simulink model "SM_Offshore_Windturbine"  (R2021a)
settings: Solver=ode4  StartTime=0.0  StopTime=par.sym.Ttot  FixedStep=par.sym.max_dt  MaxStep=par.sym.max_dt  RelTol=1e-3
model workspace: external: MATLAB File C:\Users\d053704\Desktop\MOST\Structure\CAD\CAD_DataFile.m (data not in the file)
undefined symbols (not defined in the file): par, smiData, X, Y, Z
libraries: sm_lib x50, simulink_extras x29, vrlib x18, nesl_utility x10, dspstat3 x9, sharedutil x5, eeGeneralControl x2
(part 1 of 4)
settings Model: Creator=lorenzocottura  LastModifiedBy=d053704
settings SolverCC: AlgebraicLoopSolver=LineSearch
settings DataIOCC: ReturnWorkspaceOutputs=off  TimeSaveName=TIME
settings OptimizationCC: LifeSpan=inf
settings DebuggingCC: SFMachineParentedDataDiag=warning  ArithmeticOperatorsInVariantConditions=warning
settings SFSimCC: CustomCodeUndefinedFunction=UseInterfaceOnly
settings SimscapeCC: SimscapeNormalizeSystem=off

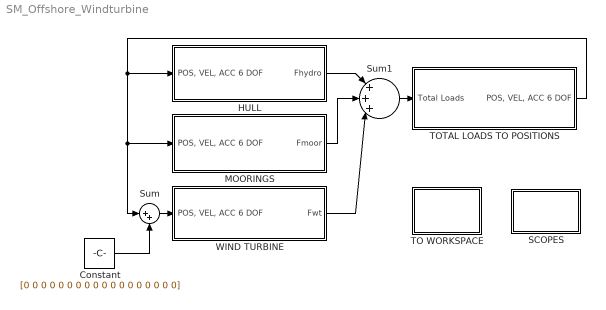
== system SM_Offshore_Windturbine ==
  Constant : Constant  Value=[0 0 0 0 0 0 0 0 0 0 0 0 0 0 0 0 0 0]
  HULL : Subsystem
  MOORINGS : Subsystem
  SCOPES : Subsystem
  Sum : Sum  Inputs=|++
  Sum1 : Sum  Inputs=|+++|
  TO WORKSPACE : Subsystem
  TOTAL LOADS TO POSITIONS : Subsystem
  WIND TURBINE : Subsystem
  wires:
  HULL/1(Fhydro) -> Sum1/1
  MOORINGS/1(Fmoor) -> Sum1/2
  WIND TURBINE/1(Fwt) -> Sum1/3
  Sum1/1 -> TOTAL LOADS TO POSITIONS/1(Total Loads)
  TOTAL LOADS TO POSITIONS/1("POS, VEL, ACC 6 DOF") -> HULL/1("POS, VEL, ACC 6 DOF"), Sum/1, MOORINGS/1("POS, VEL, ACC 6 DOF")
  Sum/1 -> WIND TURBINE/1("POS, VEL, ACC 6 DOF")
  Constant/1 -> Sum/2

== system SM_Offshore_Windturbine/HULL ==
  "POS, VEL, ACC 6 DOF" : Inport
  Add1 : Sum  Inputs=+-+-
  Hydrostatic stiffness : Subsystem
  IRR. WAVES : Subsystem
  Selector : Selector  InputPortWidth=18  IndexOptions=Index vector (dialog)  Indices=[1 2 3 4 5 6]  OutputSizes=1
  Selector1 : Selector  InputPortWidth=18  IndexOptions=Index vector (dialog)  Indices=[7 8 9 10 11 12]  OutputSizes=1
  State space model : Subsystem
  Viscous loads : Subsystem  TreatAsAtomicUnit=on
  Fhydro : Outport  VectorParamsAs1DForOutWhenUnconnected=off
  wires:
  Hydrostatic stiffness/1(Hydrostatic forces) -> Add1/2
  IRR. WAVES/1(Fw) -> Add1/1
  Selector1/1 -> State space model/1(hull_speed), Viscous loads/1(hull_speed)
  State space model/1(Radiation forces) -> Add1/4
  "POS, VEL, ACC 6 DOF"/1 -> Selector1/1, Selector/1
  Add1/1 -> Fhydro/1  "Hydrodinamic Loads"
  Viscous loads/1(Viscous forces) -> Add1/3
  Selector/1 -> Viscous loads/2(hull_position), Hydrostatic stiffness/1(hull_position)

== system SM_Offshore_Windturbine/MOORINGS ==
  "POS, VEL, ACC 6 DOF" : Inport
  6 Dof Extractor : Subsystem
  6 Dof Extractor1 : Subsystem
  6 Dof Extractor2 : Subsystem
  6 Dof Extractor3 : Subsystem
  6 Dof Extractor4 : Subsystem
  6 Dof Extractor5 : Subsystem
  Mux : Mux  Inputs=6
  n-D Lookup Table1 : Lookup_n-D  NumberOfTableDimensions=6  LookupTableObject=''  BreakpointsForDimension1=par.moor.LUT.x  BreakpointsForDimension2=par.moor.LUT.y  BreakpointsForDimension3=par.moor.LUT.z  BreakpointsForDimension4=par.moor.LUT.rx  BreakpointsForDimension5=par.moor.LUT.ry  BreakpointsForDimension6=par.moor.LUT.rz  BreakpointsForDimension1FirstPoint=10  BreakpointsForDimension2FirstPoint=10  BreakpointsForDimension1Spacing=12  BreakpointsForDimension2Spacing=12  Table=par.moor.LUT.Tx  TableDataTypeStr=Inherit: Inherit from 'Table data'  InternalRulePriority=Speed  RndMeth=Simplest  InputSameDT=on
      settings: InputPortMap=u0,u1,u2,u3,u4,u5
  n-D Lookup Table2 : Lookup_n-D  NumberOfTableDimensions=6  LookupTableObject=''  BreakpointsForDimension1=par.moor.LUT.x  BreakpointsForDimension2=par.moor.LUT.y  BreakpointsForDimension3=par.moor.LUT.z  BreakpointsForDimension4=par.moor.LUT.rx  BreakpointsForDimension5=par.moor.LUT.ry  BreakpointsForDimension6=par.moor.LUT.rz  BreakpointsForDimension1FirstPoint=10  BreakpointsForDimension2FirstPoint=10  BreakpointsForDimension1Spacing=12  BreakpointsForDimension2Spacing=12  Table=par.moor.LUT.Ty  TableDataTypeStr=Inherit: Inherit from 'Table data'  InternalRulePriority=Speed  RndMeth=Simplest  InputSameDT=on
      settings: InputPortMap=u0,u1,u2,u3,u4,u5
  n-D Lookup Table3 : Lookup_n-D  NumberOfTableDimensions=6  LookupTableObject=''  BreakpointsForDimension1=par.moor.LUT.x  BreakpointsForDimension2=par.moor.LUT.y  BreakpointsForDimension3=par.moor.LUT.z  BreakpointsForDimension4=par.moor.LUT.rx  BreakpointsForDimension5=par.moor.LUT.ry  BreakpointsForDimension6=par.moor.LUT.rz  BreakpointsForDimension1FirstPoint=10  BreakpointsForDimension2FirstPoint=10  BreakpointsForDimension1Spacing=12  BreakpointsForDimension2Spacing=12  Table=par.moor.LUT.Tz  TableDataTypeStr=Inherit: Inherit from 'Table data'  InternalRulePriority=Speed  RndMeth=Simplest  InputSameDT=on
      settings: InputPortMap=u0,u1,u2,u3,u4,u5
  n-D Lookup Table4 : Lookup_n-D  NumberOfTableDimensions=6  LookupTableObject=''  BreakpointsForDimension1=par.moor.LUT.x  BreakpointsForDimension2=par.moor.LUT.y  BreakpointsForDimension3=par.moor.LUT.z  BreakpointsForDimension4=par.moor.LUT.rx  BreakpointsForDimension5=par.moor.LUT.ry  BreakpointsForDimension6=par.moor.LUT.rz  BreakpointsForDimension1FirstPoint=10  BreakpointsForDimension2FirstPoint=10  BreakpointsForDimension1Spacing=12  BreakpointsForDimension2Spacing=12  Table=par.moor.LUT.TRx  TableDataTypeStr=Inherit: Inherit from 'Table data'  InternalRulePriority=Speed  RndMeth=Simplest  InputSameDT=on
      settings: InputPortMap=u0,u1,u2,u3,u4,u5
  n-D Lookup Table5 : Lookup_n-D  NumberOfTableDimensions=6  LookupTableObject=''  BreakpointsForDimension1=par.moor.LUT.x  BreakpointsForDimension2=par.moor.LUT.y  BreakpointsForDimension3=par.moor.LUT.z  BreakpointsForDimension4=par.moor.LUT.rx  BreakpointsForDimension5=par.moor.LUT.ry  BreakpointsForDimension6=par.moor.LUT.rz  BreakpointsForDimension1FirstPoint=10  BreakpointsForDimension2FirstPoint=10  BreakpointsForDimension1Spacing=12  BreakpointsForDimension2Spacing=12  Table=par.moor.LUT.TRy  TableDataTypeStr=Inherit: Inherit from 'Table data'  InternalRulePriority=Speed  RndMeth=Simplest  InputSameDT=on
      settings: InputPortMap=u0,u1,u2,u3,u4,u5
  n-D Lookup Table6 : Lookup_n-D  NumberOfTableDimensions=6  LookupTableObject=''  BreakpointsForDimension1=par.moor.LUT.x  BreakpointsForDimension2=par.moor.LUT.y  BreakpointsForDimension3=par.moor.LUT.z  BreakpointsForDimension4=par.moor.LUT.rx  BreakpointsForDimension5=par.moor.LUT.ry  BreakpointsForDimension6=par.moor.LUT.rz  BreakpointsForDimension1FirstPoint=10  BreakpointsForDimension2FirstPoint=10  BreakpointsForDimension1Spacing=12  BreakpointsForDimension2Spacing=12  Table=par.moor.LUT.TRz  TableDataTypeStr=Inherit: Inherit from 'Table data'  InternalRulePriority=Speed  RndMeth=Simplest  InputSameDT=on
      settings: InputPortMap=u0,u1,u2,u3,u4,u5
  Fmoor : Outport  VectorParamsAs1DForOutWhenUnconnected=off
  tag scope: MOORINGFORCES=global
  wires:
  6 Dof Extractor4/2(SWAY) -> n-D Lookup Table5/2
  n-D Lookup Table2/1 -> Mux/2  "Ty"
  6 Dof Extractor/2(SWAY) -> n-D Lookup Table1/2
  6 Dof Extractor3/6(YAW) -> n-D Lookup Table4/6
  n-D Lookup Table4/1 -> Mux/4  "TRx"
  6 Dof Extractor2/5(PITCH) -> n-D Lookup Table3/5
  6 Dof Extractor2/2(SWAY) -> n-D Lookup Table3/2
  6 Dof Extractor/1(SURGE) -> n-D Lookup Table1/1
  6 Dof Extractor5/6(YAW) -> n-D Lookup Table6/6
  n-D Lookup Table1/1 -> Mux/1  "Tx"
  6 Dof Extractor1/1(SURGE) -> n-D Lookup Table2/1
  n-D Lookup Table6/1 -> Mux/6  "TRz"
  6 Dof Extractor4/5(PITCH) -> n-D Lookup Table5/5
  6 Dof Extractor1/5(PITCH) -> n-D Lookup Table2/5
  6 Dof Extractor1/6(YAW) -> n-D Lookup Table2/6
  6 Dof Extractor2/6(YAW) -> n-D Lookup Table3/6
  6 Dof Extractor5/3(HEAVE) -> n-D Lookup Table6/3
  6 Dof Extractor/5(PITCH) -> n-D Lookup Table1/5
  n-D Lookup Table3/1 -> Mux/3  "Tz"
  6 Dof Extractor3/2(SWAY) -> n-D Lookup Table4/2
  6 Dof Extractor3/1(SURGE) -> n-D Lookup Table4/1
  6 Dof Extractor4/4(ROLL) -> n-D Lookup Table5/4
  6 Dof Extractor3/5(PITCH) -> n-D Lookup Table4/5
  6 Dof Extractor2/1(SURGE) -> n-D Lookup Table3/1
  6 Dof Extractor/4(ROLL) -> n-D Lookup Table1/4
  6 Dof Extractor3/4(ROLL) -> n-D Lookup Table4/4
  6 Dof Extractor1/2(SWAY) -> n-D Lookup Table2/2
  6 Dof Extractor/6(YAW) -> n-D Lookup Table1/6
  6 Dof Extractor1/4(ROLL) -> n-D Lookup Table2/4
  6 Dof Extractor5/4(ROLL) -> n-D Lookup Table6/4
  6 Dof Extractor1/3(HEAVE) -> n-D Lookup Table2/3
  6 Dof Extractor4/3(HEAVE) -> n-D Lookup Table5/3
  6 Dof Extractor2/4(ROLL) -> n-D Lookup Table3/4
  6 Dof Extractor4/1(SURGE) -> n-D Lookup Table5/1
  6 Dof Extractor3/3(HEAVE) -> n-D Lookup Table4/3
  6 Dof Extractor/3(HEAVE) -> n-D Lookup Table1/3
  6 Dof Extractor5/5(PITCH) -> n-D Lookup Table6/5
  6 Dof Extractor5/2(SWAY) -> n-D Lookup Table6/2
  n-D Lookup Table5/1 -> Mux/5  "TRy"
  6 Dof Extractor5/1(SURGE) -> n-D Lookup Table6/1
  6 Dof Extractor4/6(YAW) -> n-D Lookup Table5/6
  6 Dof Extractor2/3(HEAVE) -> n-D Lookup Table3/3
  Mux/1 -> Fmoor/1, [MOORINGFORCES]  "T_C"
  "POS, VEL, ACC 6 DOF"/1 -> 6 Dof Extractor4/1(6DOF), 6 Dof Extractor5/1(6DOF), 6 Dof Extractor3/1(6DOF), 6 Dof Extractor2/1(6DOF), 6 Dof Extractor1/1(6DOF), 6 Dof Extractor/1(6DOF)

== system SM_Offshore_Windturbine/SCOPES ==
  Divide1 : Product  Inputs=**
  GUIScopes : Scope  NumInputPorts=9
  Radians to Degrees4 : simulink_extras/Transformations/Radians to Degrees
  Radians to Degrees5 : simulink_extras/Transformations/Radians to Degrees
  Radians to Degrees6 : simulink_extras/Transformations/Radians to Degrees
  Selector{,1..5} (6 alike) : Selector  InputPortWidth=3  IndexOptions=Index vector (dialog)  Indices=[1]  OutputSizes=1
  W2MW1 : Gain  Gain=1e-6
  efficiency1 : Gain  Gain=0.944
  tag scope: GENPWR=global
  wires:
  [SURGE] -> Selector/1
  Selector/1 -> GUIScopes/1  "Surge [m]"
  [HEAVE] -> Selector1/1  "z"
  Selector1/1 -> GUIScopes/3  "Heave [m]"
  [SWAY] -> Selector2/1  "y"
  Selector2/1 -> GUIScopes/2  "Sway [m]"
  Radians to Degrees4/1 -> GUIScopes/4  "Roll [deg]"
  Radians to Degrees5/1 -> GUIScopes/5  "Pitch [deg]"
  Radians to Degrees6/1 -> GUIScopes/6  "Yaw [deg]"
  W2MW1/1 -> [GENPWR], GUIScopes/9  "Generator Power [MW]"
  [YAW] -> Selector4/1  "ry"
  Selector4/1 -> Radians to Degrees6/1
  Selector5/1 -> Radians to Degrees5/1
  Selector3/1 -> Radians to Degrees4/1
  [ROLL] -> Selector3/1  "ry"
  [PITCH] -> Selector5/1  "ry"
  [BlPITCH] -> GUIScopes/8  "Blade Pitch [deg]"
  [GENSPD] -> GUIScopes/7  "Generator Speed [rpm]"
  [Speed] -> Divide1/2
  [GENTRQ] -> Divide1/1  "GENTRQ"
  efficiency1/1 -> W2MW1/1
  Divide1/1 -> efficiency1/1

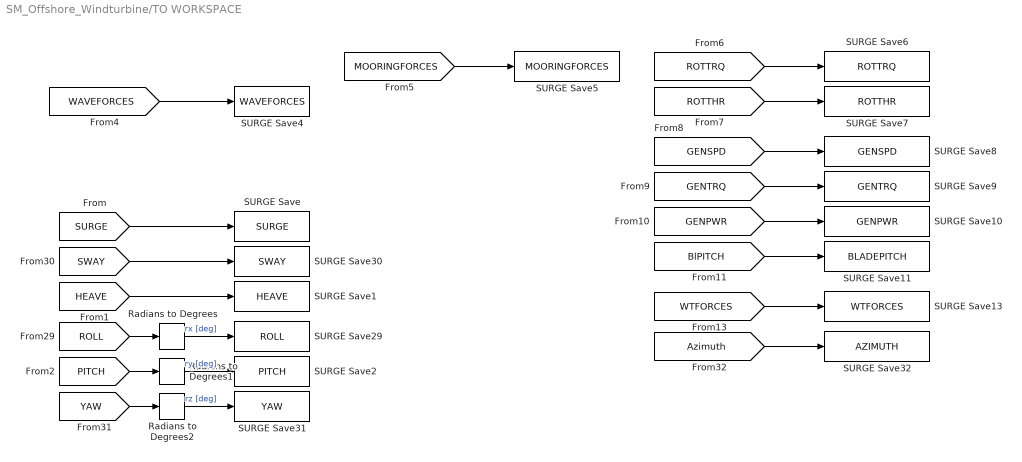
== system SM_Offshore_Windturbine/TO WORKSPACE ==
  Radians to Degrees : simulink_extras/Transformations/Radians to Degrees
  Radians to Degrees1 : simulink_extras/Transformations/Radians to Degrees
  Radians to Degrees2 : simulink_extras/Transformations/Radians to Degrees
  SURGE Save : ToWorkspace  VariableName=SURGE  SampleTime=-1
  SURGE Save1 : ToWorkspace  VariableName=HEAVE  SampleTime=-1
  SURGE Save10 : ToWorkspace  VariableName=GENPWR  SampleTime=-1
  SURGE Save11 : ToWorkspace  VariableName=BLADEPITCH  SampleTime=-1
  SURGE Save13 : ToWorkspace  VariableName=WTFORCES  SampleTime=-1
  SURGE Save2 : ToWorkspace  VariableName=PITCH  SampleTime=-1
  SURGE Save29 : ToWorkspace  VariableName=ROLL  SampleTime=-1
  SURGE Save30 : ToWorkspace  VariableName=SWAY  SampleTime=-1
  SURGE Save31 : ToWorkspace  VariableName=YAW  SampleTime=-1
  SURGE Save32 : ToWorkspace  VariableName=AZIMUTH  SampleTime=-1
  SURGE Save4 : ToWorkspace  VariableName=WAVEFORCES  SampleTime=-1
  SURGE Save5 : ToWorkspace  VariableName=MOORINGFORCES  SampleTime=-1
  SURGE Save6 : ToWorkspace  VariableName=ROTTRQ  SampleTime=-1
  SURGE Save7 : ToWorkspace  VariableName=ROTTHR  SampleTime=-1
  SURGE Save8 : ToWorkspace  VariableName=GENSPD  SampleTime=-1
  SURGE Save9 : ToWorkspace  VariableName=GENTRQ  SampleTime=-1
  wires:
  [SURGE] -> SURGE Save/1
  [HEAVE] -> SURGE Save1/1
  [PITCH] -> Radians to Degrees1/1
  [WAVEFORCES] -> SURGE Save4/1
  [MOORINGFORCES] -> SURGE Save5/1
  [ROTTRQ] -> SURGE Save6/1
  [ROTTHR] -> SURGE Save7/1
  [GENSPD] -> SURGE Save8/1
  [GENTRQ] -> SURGE Save9/1
  [GENPWR] -> SURGE Save10/1
  [BlPITCH] -> SURGE Save11/1
  [WTFORCES] -> SURGE Save13/1
  [ROLL] -> Radians to Degrees/1
  [YAW] -> Radians to Degrees2/1
  [SWAY] -> SURGE Save30/1
  [Azimuth] -> SURGE Save32/1
  Radians to Degrees/1 -> SURGE Save29/1  "rx [deg]"
  Radians to Degrees1/1 -> SURGE Save2/1  "ry [deg]"
  Radians to Degrees2/1 -> SURGE Save31/1  "rz [deg]"

== system SM_Offshore_Windturbine/TOTAL LOADS TO POSITIONS ==
  Total Loads : Inport
  "6 Dof Extractor TO SCOPES " : Subsystem
  Add : Sum  Inputs=-+-
  Added mass matrix : Constant  Value=par.hull.TDM.Ainf
  Gravity & Restoring moment : Subsystem
  Integrator : Integrator
  Integrator2 : Integrator
  Matrix Divide : Product  Inputs=/*  Multiplication=Matrix(*)
  Memory1 : Memory
  Memory2 : Memory
  Memory3 : Memory
  Mux : Mux  Inputs=3
  "Non linear loads " : Subsystem
  Sum : Sum
  Variable mass matrix1 : ModelReference  ModelNameDialog=Variable_mass_matrix.slxp  ModelReferenceVersion=5.19  CopyOfModelProtected=on
  "POS, VEL, ACC 6 DOF" : Outport  VectorParamsAs1DForOutWhenUnconnected=off
  wires:
  Integrator2/1 -> Memory2/1  "Position"
  Add/1 -> Matrix Divide/2
  Matrix Divide/1 -> Integrator/1, Memory3/1  "Acceleration"
  Variable mass matrix1/1 -> "Non linear loads "/1(MassMatrix), Sum/2, Gravity & Restoring moment/1(MassMatrix)
  "Non linear loads "/1(Non_linear) -> Add/3
  Mux/1 -> "POS, VEL, ACC 6 DOF"/1, "6 Dof Extractor TO SCOPES "/1(6DOF)
  Integrator/1 -> Integrator2/1, Memory1/1
  Memory2/1 -> Variable mass matrix1/1, Mux/1
  Memory1/1 -> "Non linear loads "/2(hull_speed), Mux/2
  Memory3/1 -> Mux/3
  Gravity & Restoring moment/1(Gravity & Restoring moment) -> Add/1
  Added mass matrix/1 -> Sum/1
  Sum/1 -> Matrix Divide/1
  Total Loads/1 -> Add/2

== system SM_Offshore_Windturbine/WIND TURBINE ==
  "POS, VEL, ACC 6 DOF" : Inport
  BODIES MOTIONS : Subsystem
  CONTROL SYSTEM : Subsystem
  N : Gain  Gain=par.WT.prop.Ngear
  "N " : Gain  Gain=par.WT.prop.Ngear
  ROTOR LOADS : Subsystem
  Fwt : Outport  VectorParamsAs1DForOutWhenUnconnected=off
  wires:
  ROTOR LOADS/1(WT Forces) -> Fwt/1
  CONTROL SYSTEM/1(Blade pitch) -> ROTOR LOADS/1(Blade pitch in), BODIES MOTIONS/1(Blade Pitch)
  CONTROL SYSTEM/3(Tg) -> "N "/1
  N/1 -> CONTROL SYSTEM/2(Generator speed)
  ROTOR LOADS/2(RotorTorque) -> BODIES MOTIONS/2(Rotor Torque)
  "N "/1 -> ROTOR LOADS/4(Control torque), BODIES MOTIONS/4(Control Torque)
  BODIES MOTIONS/1(Rotor Speed) -> ROTOR LOADS/2(Rotor speed), N/1
  "POS, VEL, ACC 6 DOF"/1 -> CONTROL SYSTEM/1(6 DOF)
  CONTROL SYSTEM/2(6 DOF nac) -> BODIES MOTIONS/3(6 DOF), ROTOR LOADS/3(6 DOF)
  ROTOR LOADS/3(Wind Direct) -> CONTROL SYSTEM/3(Wind direction)

== system SM_Offshore_Windturbine/HULL/Hydrostatic stiffness ==
  hull_position : Inport
  Constant : Constant  Value=[0 0 par.hull.GEOM.V0*par.hull.ENV.rho_w*9.80665 0 0 0]
  Hydrostatic stiffness : Constant  Value=par.hull.FDA.hydrostatic.K
  Product2 : Product  Multiplication=Matrix(*)  RndMeth=Zero
  Sum1 : Sum  Inputs=|+-
  Hydrostatic forces : Outport  VectorParamsAs1DForOutWhenUnconnected=off
  wires:
  Sum1/1 -> Hydrostatic forces/1
  Constant/1 -> Sum1/2
  Product2/1 -> Sum1/1
  Hydrostatic stiffness/1 -> Product2/1
  hull_position/1 -> Product2/2

== system SM_Offshore_Windturbine/HULL/IRR. WAVES ==
  Excitation forces : FromWorkspace  VariableName=[par.wave.TIME,par.wave.forces.TAU]
  Fw : Outport  VectorParamsAs1DForOutWhenUnconnected=off
  tag scope: WAVEFORCES=global
  wires:
  Excitation forces/1 -> [WAVEFORCES], Fw/1

== system SM_Offshore_Windturbine/HULL/State space model ==
  hull_speed : Inport
  Demux : Demux  Outputs=6
  Mux : Mux  Inputs=6
  State-Space1 : StateSpace  A=par.hull.TDM.(DOFs).Ass  B=par.hull.TDM.(DOFs).Bss  C=par.hull.TDM.(DOFs).Css  D=par.hull.TDM.(DOFs).Dss  InitialCondition=0  mask{DOFs='y'}
      mask prompts: DOFs "Degree of freedom selection (e.g. 'x_ry', 'x'; include apostrophes)"
      mask help:
      | State-space model:
      |    dx/dt = Ax + Bu
      |            y = Cx + Du
      mask Display:
      | color('black')
      | 
      | if isempty(findstr(DOFs,'_'))
      |     in = DOFs;
      | else
      |     in = DOFs(1:findstr(DOFs,'_')-1);
      | end
      | 
      | port_label('input',1,in)
      | port_label('output',1,['F_{r,', strrep(DOFs,'_','-'), '}'],'texmode','on')
      | 
      | 
      | disp(['x'' = Ax + Bu' 10 'y = Cx + Du'],'texmode','on')
      | % text(0.5, 0, DOFs, 'horizontalAlignment', 'center', 'verticalAlignment', 'bottom')
  State-Space10 : StateSpace  A=par.hull.TDM.(DOFs).Ass  B=par.hull.TDM.(DOFs).Bss  C=par.hull.TDM.(DOFs).Css  D=par.hull.TDM.(DOFs).Dss  InitialCondition=0  mask{DOFs='rz'}
      mask prompts: DOFs "Degree of freedom selection (e.g. 'x_ry', 'x'; include apostrophes)"
      mask help:
      | State-space model:
      |    dx/dt = Ax + Bu
      |            y = Cx + Du
      mask Display:
      | color('black')
      | 
      | if isempty(findstr(DOFs,'_'))
      |     in = DOFs;
      | else
      |     in = DOFs(1:findstr(DOFs,'_')-1);
      | end
      | 
      | port_label('input',1,in)
      | port_label('output',1,['F_{r,', strrep(DOFs,'_','-'), '}'],'texmode','on')
      | 
      | 
      | disp(['x'' = Ax + Bu' 10 'y = Cx + Du'],'texmode','on')
      | % text(0.5, 0, DOFs, 'horizontalAlignment', 'center', 'verticalAlignment', 'bottom')
  State-Space2 : StateSpace  A=par.hull.TDM.(DOFs).Ass  B=par.hull.TDM.(DOFs).Bss  C=par.hull.TDM.(DOFs).Css  D=par.hull.TDM.(DOFs).Dss  InitialCondition=0  mask{DOFs='x'}
      mask prompts: DOFs "Degree of freedom selection (e.g. 'x_ry', 'x'; include apostrophes)"
      mask help:
      | State-space model:
      |    dx/dt = Ax + Bu
      |            y = Cx + Du
      mask Display:
      | color('black')
      | 
      | if isempty(findstr(DOFs,'_'))
      |     in = DOFs;
      | else
      |     in = DOFs(1:findstr(DOFs,'_')-1);
      | end
      | 
      | port_label('input',1,in)
      | port_label('output',1,['F_{r,', strrep(DOFs,'_','-'), '}'],'texmode','on')
      | 
      | 
      | disp(['x'' = Ax + Bu' 10 'y = Cx + Du'],'texmode','on')
  State-Space3 : StateSpace  A=par.hull.TDM.(DOFs).Ass  B=par.hull.TDM.(DOFs).Bss  C=par.hull.TDM.(DOFs).Css  D=par.hull.TDM.(DOFs).Dss  InitialCondition=0  mask{DOFs='ry_x'}
      mask prompts: DOFs "Degree of freedom selection (e.g. 'x_ry', 'x'; include apostrophes)"
      mask help:
      | State-space model:
      |    dx/dt = Ax + Bu
      |            y = Cx + Du
      mask Display:
      | color('black')
      | 
      | if isempty(findstr(DOFs,'_'))
      |     in = DOFs;
      | else
      |     in = DOFs(1:findstr(DOFs,'_')-1);
      | end
      | 
      | port_label('input',1,in)
      | port_label('output',1,['F_{r,', strrep(DOFs,'_','-'), '}'],'texmode','on')
      | 
      | 
      | disp(['x'' = Ax + Bu' 10 'y = Cx + Du'],'texmode','on')
      | % text(0.5, 0, DOFs, 'horizontalAlignment', 'center', 'verticalAlignment', 'bottom')
  State-Space4 : StateSpace  A=par.hull.TDM.(DOFs).Ass  B=par.hull.TDM.(DOFs).Bss  C=par.hull.TDM.(DOFs).Css  D=par.hull.TDM.(DOFs).Dss  InitialCondition=0  mask{DOFs='rx'}
      mask prompts: DOFs "Degree of freedom selection (e.g. 'x_ry', 'x'; include apostrophes)"
      mask help:
      | State-space model:
      |    dx/dt = Ax + Bu
      |            y = Cx + Du
      mask Display:
      | color('black')
      | 
      | if isempty(findstr(DOFs,'_'))
      |     in = DOFs;
      | else
      |     in = DOFs(1:findstr(DOFs,'_')-1);
      | end
      | 
      | port_label('input',1,in)
      | port_label('output',1,['F_{r,', strrep(DOFs,'_','-'), '}'],'texmode','on')
      | 
      | 
      | disp(['x'' = Ax + Bu' 10 'y = Cx + Du'],'texmode','on')
      | % text(0.5, 0, DOFs, 'horizontalAlignment', 'center', 'verticalAlignment', 'bottom')
  State-Space5 : StateSpace  A=par.hull.TDM.(DOFs).Ass  B=par.hull.TDM.(DOFs).Bss  C=par.hull.TDM.(DOFs).Css  D=par.hull.TDM.(DOFs).Dss  InitialCondition=0  mask{DOFs='z'}
      mask prompts: DOFs "Degree of freedom selection (e.g. 'x_ry', 'x'; include apostrophes)"
      mask help:
      | State-space model:
      |    dx/dt = Ax + Bu
      |            y = Cx + Du
      mask Display:
      | color('black')
      | 
      | if isempty(findstr(DOFs,'_'))
      |     in = DOFs;
      | else
      |     in = DOFs(1:findstr(DOFs,'_')-1);
      | end
      | 
      | port_label('input',1,in)
      | port_label('output',1,['F_{r,', strrep(DOFs,'_','-'), '}'],'texmode','on')
      | 
      | 
      | disp(['x'' = Ax + Bu' 10 'y = Cx + Du'],'texmode','on')
      | % text(0.5, 0, DOFs, 'horizontalAlignment', 'center', 'verticalAlignment', 'bottom')
  State-Space6 : StateSpace  A=par.hull.TDM.(DOFs).Ass  B=par.hull.TDM.(DOFs).Bss  C=par.hull.TDM.(DOFs).Css  D=par.hull.TDM.(DOFs).Dss  InitialCondition=0  mask{DOFs='x_ry'}
      mask prompts: DOFs "Degree of freedom selection (e.g. 'x_ry', 'x'; include apostrophes)"
      mask help:
      | State-space model:
      |    dx/dt = Ax + Bu
      |            y = Cx + Du
      mask Display:
      | color('black')
      | 
      | if isempty(findstr(DOFs,'_'))
      |     in = DOFs;
      | else
      |     in = DOFs(1:findstr(DOFs,'_')-1);
      | end
      | 
      | port_label('input',1,in)
      | port_label('output',1,['F_{r,', strrep(DOFs,'_','-'), '}'],'texmode','on')
      | 
      | 
      | disp(['x'' = Ax + Bu' 10 'y = Cx + Du'],'texmode','on')
      | % text(0.5, 0, DOFs, 'horizontalAlignment', 'center', 'verticalAlignment', 'bottom')
  State-Space7 : StateSpace  A=par.hull.TDM.(DOFs).Ass  B=par.hull.TDM.(DOFs).Bss  C=par.hull.TDM.(DOFs).Css  D=par.hull.TDM.(DOFs).Dss  InitialCondition=0  mask{DOFs='rx_y'}
      mask prompts: DOFs "Degree of freedom selection (e.g. 'x_ry', 'x'; include apostrophes)"
      mask help:
      | State-space model:
      |    dx/dt = Ax + Bu
      |            y = Cx + Du
      mask Display:
      | color('black')
      | 
      | if isempty(findstr(DOFs,'_'))
      |     in = DOFs;
      | else
      |     in = DOFs(1:findstr(DOFs,'_')-1);
      | end
      | 
      | port_label('input',1,in)
      | port_label('output',1,['F_{r,', strrep(DOFs,'_','-'), '}'],'texmode','on')
      | 
      | 
      | disp(['x'' = Ax + Bu' 10 'y = Cx + Du'],'texmode','on')
      | % text(0.5, 0, DOFs, 'horizontalAlignment', 'center', 'verticalAlignment', 'bottom')
  State-Space8 : StateSpace  A=par.hull.TDM.(DOFs).Ass  B=par.hull.TDM.(DOFs).Bss  C=par.hull.TDM.(DOFs).Css  D=par.hull.TDM.(DOFs).Dss  InitialCondition=0  mask{DOFs='ry'}
      mask prompts: DOFs "Degree of freedom selection (e.g. 'x_ry', 'x'; include apostrophes)"
      mask help:
      | State-space model:
      |    dx/dt = Ax + Bu
      |            y = Cx + Du
      mask Display:
      | color('black')
      | 
      | if isempty(findstr(DOFs,'_'))
      |     in = DOFs;
      | else
      |     in = DOFs(1:findstr(DOFs,'_')-1);
      | end
      | 
      | port_label('input',1,in)
      | port_label('output',1,['F_{r,', strrep(DOFs,'_','-'), '}'],'texmode','on')
      | 
      | 
      | disp(['x'' = Ax + Bu' 10 'y = Cx + Du'],'texmode','on')
      | % text(0.5, 0, DOFs, 'horizontalAlignment', 'center', 'verticalAlignment', 'bottom')
  State-Space9 : StateSpace  A=par.hull.TDM.(DOFs).Ass  B=par.hull.TDM.(DOFs).Bss  C=par.hull.TDM.(DOFs).Css  D=par.hull.TDM.(DOFs).Dss  InitialCondition=0  mask{DOFs='y_rx'}
      mask prompts: DOFs "Degree of freedom selection (e.g. 'x_ry', 'x'; include apostrophes)"
      mask help:
      | State-space model:
      |    dx/dt = Ax + Bu
      |            y = Cx + Du
      mask Display:
      | color('black')
      | 
      | if isempty(findstr(DOFs,'_'))
      |     in = DOFs;
      | else
      |     in = DOFs(1:findstr(DOFs,'_')-1);
      | end
      | 
      | port_label('input',1,in)
      | port_label('output',1,['F_{r,', strrep(DOFs,'_','-'), '}'],'texmode','on')
      | 
      | 
      | disp(['x'' = Ax + Bu' 10 'y = Cx + Du'],'texmode','on')
      | % text(0.5, 0, DOFs, 'horizontalAlignment', 'center', 'verticalAlignment', 'bottom')
  Sum{,1..3} (4 alike) : Sum  Inputs=|++
  Radiation forces : Outport  VectorParamsAs1DForOutWhenUnconnected=off
  wires:
  Demux/3 -> State-Space5/1
  Demux/5 -> State-Space8/1, State-Space3/1
  Demux/6 -> State-Space10/1
  Demux/1 -> State-Space6/1, State-Space2/1
  State-Space3/1 -> Sum/2
  State-Space2/1 -> Sum/1
  Sum1/1 -> Mux/5
  Sum/1 -> Mux/1
  State-Space5/1 -> Mux/3
  State-Space1/1 -> Sum2/1
  State-Space4/1 -> Sum3/1
  Demux/4 -> State-Space4/1, State-Space7/1
  State-Space7/1 -> Sum2/2
  State-Space6/1 -> Sum1/2
  State-Space8/1 -> Sum1/1
  State-Space9/1 -> Sum3/2
  Demux/2 -> State-Space9/1, State-Space1/1
  Sum2/1 -> Mux/2
  Sum3/1 -> Mux/4
  State-Space10/1 -> Mux/6
  Mux/1 -> Radiation forces/1
  hull_speed/1 -> Demux/1

== system SM_Offshore_Windturbine/HULL/Viscous loads ==
  hull_speed : Inport
  hull_position : Inport  Port=2
  Added damping loads : Subsystem
  Constant : Constant  Value=par.hull.drag.Cd
  Constant1 : Constant  Value=par.hull.drag.D
  Constant2 : Constant  Value=par.hull.drag.z
  Integration_Drag : ModelReference  ModelNameDialog=Integration_Drag.slxp  ModelReferenceVersion=5.19  CopyOfModelProtected=on
  Subsystem1 : Subsystem
  Sum : Sum  Inputs=-+|
  Viscous forces : Outport  VectorParamsAs1DForOutWhenUnconnected=off
  wires:
  Sum/1 -> Viscous forces/1
  Constant1/1 -> Integration_Drag/4
  Constant2/1 -> Integration_Drag/5
  hull_speed/1 -> Subsystem1/1(hull_speed), Added damping loads/1(hull_speed)
  Integration_Drag/1 -> Sum/2
  Added damping loads/1(Added Damping) -> Sum/1
  hull_position/1 -> Subsystem1/2(hull_position)
  Subsystem1/1(Vx) -> Integration_Drag/1
  Subsystem1/2(Vy) -> Integration_Drag/2
  Constant/1 -> Integration_Drag/3

== system SM_Offshore_Windturbine/MOORINGS/6 Dof Extractor ==
  note: SURGE
  note: HEAVE
  note: PITCH
  6DOF : Inport  PortDimensions=18
  Radians to Degrees : simulink_extras/Transformations/Radians to Degrees
  Radians to Degrees1 : simulink_extras/Transformations/Radians to Degrees
  Radians to Degrees2 : simulink_extras/Transformations/Radians to Degrees
  rx,rxdot,rxdotdot : Selector  InputPortWidth=18  IndexOptions=Index vector (dialog)  Indices=4  OutputSizes=1
  ry,rydot,rydotdot : Selector  InputPortWidth=18  IndexOptions=Index vector (dialog)  Indices=5  OutputSizes=1
  "rz,rzdot,rzdotdot " : Selector  InputPortWidth=18  IndexOptions=Index vector (dialog)  Indices=6  OutputSizes=1
  x,xdot,xdotdot : Selector  InputPortWidth=18  IndexOptions=Index vector (dialog)  Indices=1  OutputSizes=1
  y,ydot,ydotdot : Selector  InputPortWidth=18  IndexOptions=Index vector (dialog)  Indices=2  OutputSizes=1
  z,zdot,zdotdot : Selector  InputPortWidth=18  IndexOptions=Index vector (dialog)  Indices=3  OutputSizes=1
  SURGE : Outport  VectorParamsAs1DForOutWhenUnconnected=off
  SWAY : Outport  Port=2  VectorParamsAs1DForOutWhenUnconnected=off
  HEAVE : Outport  Port=3  VectorParamsAs1DForOutWhenUnconnected=off
  ROLL : Outport  Port=4  VectorParamsAs1DForOutWhenUnconnected=off
  PITCH : Outport  Port=5  VectorParamsAs1DForOutWhenUnconnected=off
  YAW : Outport  Port=6  VectorParamsAs1DForOutWhenUnconnected=off
  wires:
  Radians to Degrees2/1 -> YAW/1
  Radians to Degrees1/1 -> PITCH/1
  Radians to Degrees/1 -> ROLL/1
  6DOF/1 -> z,zdot,zdotdot/1, x,xdot,xdotdot/1, y,ydot,ydotdot/1, ry,rydot,rydotdot/1, "rz,rzdot,rzdotdot "/1, rx,rxdot,rxdotdot/1
  "rz,rzdot,rzdotdot "/1 -> Radians to Degrees2/1
  ry,rydot,rydotdot/1 -> Radians to Degrees1/1
  rx,rxdot,rxdotdot/1 -> Radians to Degrees/1
  z,zdot,zdotdot/1 -> HEAVE/1
  y,ydot,ydotdot/1 -> SWAY/1
  x,xdot,xdotdot/1 -> SURGE/1

== system SM_Offshore_Windturbine/MOORINGS/6 Dof Extractor1 ==
  note: PITCH
  note: HEAVE
  note: SURGE
  6DOF : Inport  PortDimensions=18
  Radians to Degrees : simulink_extras/Transformations/Radians to Degrees
  Radians to Degrees1 : simulink_extras/Transformations/Radians to Degrees
  Radians to Degrees2 : simulink_extras/Transformations/Radians to Degrees
  rx,rxdot,rxdotdot : Selector  InputPortWidth=18  IndexOptions=Index vector (dialog)  Indices=4  OutputSizes=1
  ry,rydot,rydotdot : Selector  InputPortWidth=18  IndexOptions=Index vector (dialog)  Indices=5  OutputSizes=1
  "rz,rzdot,rzdotdot " : Selector  InputPortWidth=18  IndexOptions=Index vector (dialog)  Indices=6  OutputSizes=1
  x,xdot,xdotdot : Selector  InputPortWidth=18  IndexOptions=Index vector (dialog)  Indices=1  OutputSizes=1
  y,ydot,ydotdot : Selector  InputPortWidth=18  IndexOptions=Index vector (dialog)  Indices=2  OutputSizes=1
  z,zdot,zdotdot : Selector  InputPortWidth=18  IndexOptions=Index vector (dialog)  Indices=3  OutputSizes=1
  SURGE : Outport  VectorParamsAs1DForOutWhenUnconnected=off
  SWAY : Outport  Port=2  VectorParamsAs1DForOutWhenUnconnected=off
  HEAVE : Outport  Port=3  VectorParamsAs1DForOutWhenUnconnected=off
  ROLL : Outport  Port=4  VectorParamsAs1DForOutWhenUnconnected=off
  PITCH : Outport  Port=5  VectorParamsAs1DForOutWhenUnconnected=off
  YAW : Outport  Port=6  VectorParamsAs1DForOutWhenUnconnected=off
  wires:
  x,xdot,xdotdot/1 -> SURGE/1
  y,ydot,ydotdot/1 -> SWAY/1
  z,zdot,zdotdot/1 -> HEAVE/1
  rx,rxdot,rxdotdot/1 -> Radians to Degrees/1
  ry,rydot,rydotdot/1 -> Radians to Degrees1/1
  "rz,rzdot,rzdotdot "/1 -> Radians to Degrees2/1
  6DOF/1 -> rx,rxdot,rxdotdot/1, "rz,rzdot,rzdotdot "/1, ry,rydot,rydotdot/1, y,ydot,ydotdot/1, x,xdot,xdotdot/1, z,zdot,zdotdot/1
  Radians to Degrees/1 -> ROLL/1
  Radians to Degrees1/1 -> PITCH/1
  Radians to Degrees2/1 -> YAW/1

== system SM_Offshore_Windturbine/MOORINGS/6 Dof Extractor2 ==
  note: SURGE
  note: HEAVE
  note: PITCH
  6DOF : Inport  PortDimensions=18
  Radians to Degrees : simulink_extras/Transformations/Radians to Degrees
  Radians to Degrees1 : simulink_extras/Transformations/Radians to Degrees
  Radians to Degrees2 : simulink_extras/Transformations/Radians to Degrees
  rx,rxdot,rxdotdot : Selector  InputPortWidth=18  IndexOptions=Index vector (dialog)  Indices=4  OutputSizes=1
  ry,rydot,rydotdot : Selector  InputPortWidth=18  IndexOptions=Index vector (dialog)  Indices=5  OutputSizes=1
  "rz,rzdot,rzdotdot " : Selector  InputPortWidth=18  IndexOptions=Index vector (dialog)  Indices=6  OutputSizes=1
  x,xdot,xdotdot : Selector  InputPortWidth=18  IndexOptions=Index vector (dialog)  Indices=1  OutputSizes=1
  y,ydot,ydotdot : Selector  InputPortWidth=18  IndexOptions=Index vector (dialog)  Indices=2  OutputSizes=1
  z,zdot,zdotdot : Selector  InputPortWidth=18  IndexOptions=Index vector (dialog)  Indices=3  OutputSizes=1
  SURGE : Outport  VectorParamsAs1DForOutWhenUnconnected=off
  SWAY : Outport  Port=2  VectorParamsAs1DForOutWhenUnconnected=off
  HEAVE : Outport  Port=3  VectorParamsAs1DForOutWhenUnconnected=off
  ROLL : Outport  Port=4  VectorParamsAs1DForOutWhenUnconnected=off
  PITCH : Outport  Port=5  VectorParamsAs1DForOutWhenUnconnected=off
  YAW : Outport  Port=6  VectorParamsAs1DForOutWhenUnconnected=off
  wires:
  Radians to Degrees2/1 -> YAW/1
  Radians to Degrees1/1 -> PITCH/1
  Radians to Degrees/1 -> ROLL/1
  6DOF/1 -> z,zdot,zdotdot/1, x,xdot,xdotdot/1, y,ydot,ydotdot/1, ry,rydot,rydotdot/1, "rz,rzdot,rzdotdot "/1, rx,rxdot,rxdotdot/1
  "rz,rzdot,rzdotdot "/1 -> Radians to Degrees2/1
  ry,rydot,rydotdot/1 -> Radians to Degrees1/1
  rx,rxdot,rxdotdot/1 -> Radians to Degrees/1
  z,zdot,zdotdot/1 -> HEAVE/1
  y,ydot,ydotdot/1 -> SWAY/1
  x,xdot,xdotdot/1 -> SURGE/1

== system SM_Offshore_Windturbine/MOORINGS/6 Dof Extractor3 ==
  note: PITCH
  note: HEAVE
  note: SURGE
  6DOF : Inport  PortDimensions=18
  Radians to Degrees : simulink_extras/Transformations/Radians to Degrees
  Radians to Degrees1 : simulink_extras/Transformations/Radians to Degrees
  Radians to Degrees2 : simulink_extras/Transformations/Radians to Degrees
  rx,rxdot,rxdotdot : Selector  InputPortWidth=18  IndexOptions=Index vector (dialog)  Indices=4  OutputSizes=1
  ry,rydot,rydotdot : Selector  InputPortWidth=18  IndexOptions=Index vector (dialog)  Indices=5  OutputSizes=1
  "rz,rzdot,rzdotdot " : Selector  InputPortWidth=18  IndexOptions=Index vector (dialog)  Indices=6  OutputSizes=1
  x,xdot,xdotdot : Selector  InputPortWidth=18  IndexOptions=Index vector (dialog)  Indices=1  OutputSizes=1
  y,ydot,ydotdot : Selector  InputPortWidth=18  IndexOptions=Index vector (dialog)  Indices=2  OutputSizes=1
  z,zdot,zdotdot : Selector  InputPortWidth=18  IndexOptions=Index vector (dialog)  Indices=3  OutputSizes=1
  SURGE : Outport  VectorParamsAs1DForOutWhenUnconnected=off
  SWAY : Outport  Port=2  VectorParamsAs1DForOutWhenUnconnected=off
  HEAVE : Outport  Port=3  VectorParamsAs1DForOutWhenUnconnected=off
  ROLL : Outport  Port=4  VectorParamsAs1DForOutWhenUnconnected=off
  PITCH : Outport  Port=5  VectorParamsAs1DForOutWhenUnconnected=off
  YAW : Outport  Port=6  VectorParamsAs1DForOutWhenUnconnected=off
  wires:
  x,xdot,xdotdot/1 -> SURGE/1
  y,ydot,ydotdot/1 -> SWAY/1
  z,zdot,zdotdot/1 -> HEAVE/1
  rx,rxdot,rxdotdot/1 -> Radians to Degrees/1
  ry,rydot,rydotdot/1 -> Radians to Degrees1/1
  "rz,rzdot,rzdotdot "/1 -> Radians to Degrees2/1
  6DOF/1 -> rx,rxdot,rxdotdot/1, "rz,rzdot,rzdotdot "/1, ry,rydot,rydotdot/1, y,ydot,ydotdot/1, x,xdot,xdotdot/1, z,zdot,zdotdot/1
  Radians to Degrees/1 -> ROLL/1
  Radians to Degrees1/1 -> PITCH/1
  Radians to Degrees2/1 -> YAW/1

== system SM_Offshore_Windturbine/MOORINGS/6 Dof Extractor4 ==
  note: SURGE
  note: HEAVE
  note: PITCH
  6DOF : Inport  PortDimensions=18
  Radians to Degrees : simulink_extras/Transformations/Radians to Degrees
  Radians to Degrees1 : simulink_extras/Transformations/Radians to Degrees
  Radians to Degrees2 : simulink_extras/Transformations/Radians to Degrees
  rx,rxdot,rxdotdot : Selector  InputPortWidth=18  IndexOptions=Index vector (dialog)  Indices=4  OutputSizes=1
  ry,rydot,rydotdot : Selector  InputPortWidth=18  IndexOptions=Index vector (dialog)  Indices=5  OutputSizes=1
  "rz,rzdot,rzdotdot " : Selector  InputPortWidth=18  IndexOptions=Index vector (dialog)  Indices=6  OutputSizes=1
  x,xdot,xdotdot : Selector  InputPortWidth=18  IndexOptions=Index vector (dialog)  Indices=1  OutputSizes=1
  y,ydot,ydotdot : Selector  InputPortWidth=18  IndexOptions=Index vector (dialog)  Indices=2  OutputSizes=1
  z,zdot,zdotdot : Selector  InputPortWidth=18  IndexOptions=Index vector (dialog)  Indices=3  OutputSizes=1
  SURGE : Outport  VectorParamsAs1DForOutWhenUnconnected=off
  SWAY : Outport  Port=2  VectorParamsAs1DForOutWhenUnconnected=off
  HEAVE : Outport  Port=3  VectorParamsAs1DForOutWhenUnconnected=off
  ROLL : Outport  Port=4  VectorParamsAs1DForOutWhenUnconnected=off
  PITCH : Outport  Port=5  VectorParamsAs1DForOutWhenUnconnected=off
  YAW : Outport  Port=6  VectorParamsAs1DForOutWhenUnconnected=off
  wires:
  Radians to Degrees2/1 -> YAW/1
  Radians to Degrees1/1 -> PITCH/1
  Radians to Degrees/1 -> ROLL/1
  6DOF/1 -> z,zdot,zdotdot/1, x,xdot,xdotdot/1, y,ydot,ydotdot/1, ry,rydot,rydotdot/1, "rz,rzdot,rzdotdot "/1, rx,rxdot,rxdotdot/1
  "rz,rzdot,rzdotdot "/1 -> Radians to Degrees2/1
  ry,rydot,rydotdot/1 -> Radians to Degrees1/1
  rx,rxdot,rxdotdot/1 -> Radians to Degrees/1
  z,zdot,zdotdot/1 -> HEAVE/1
  y,ydot,ydotdot/1 -> SWAY/1
  x,xdot,xdotdot/1 -> SURGE/1

== system SM_Offshore_Windturbine/MOORINGS/6 Dof Extractor5 ==
  note: PITCH
  note: HEAVE
  note: SURGE
  6DOF : Inport  PortDimensions=18
  Radians to Degrees : simulink_extras/Transformations/Radians to Degrees
  Radians to Degrees1 : simulink_extras/Transformations/Radians to Degrees
  Radians to Degrees2 : simulink_extras/Transformations/Radians to Degrees
  rx,rxdot,rxdotdot : Selector  InputPortWidth=18  IndexOptions=Index vector (dialog)  Indices=4  OutputSizes=1
  ry,rydot,rydotdot : Selector  InputPortWidth=18  IndexOptions=Index vector (dialog)  Indices=5  OutputSizes=1
  "rz,rzdot,rzdotdot " : Selector  InputPortWidth=18  IndexOptions=Index vector (dialog)  Indices=6  OutputSizes=1
  x,xdot,xdotdot : Selector  InputPortWidth=18  IndexOptions=Index vector (dialog)  Indices=1  OutputSizes=1
  y,ydot,ydotdot : Selector  InputPortWidth=18  IndexOptions=Index vector (dialog)  Indices=2  OutputSizes=1
  z,zdot,zdotdot : Selector  InputPortWidth=18  IndexOptions=Index vector (dialog)  Indices=3  OutputSizes=1
  SURGE : Outport  VectorParamsAs1DForOutWhenUnconnected=off
  SWAY : Outport  Port=2  VectorParamsAs1DForOutWhenUnconnected=off
  HEAVE : Outport  Port=3  VectorParamsAs1DForOutWhenUnconnected=off
  ROLL : Outport  Port=4  VectorParamsAs1DForOutWhenUnconnected=off
  PITCH : Outport  Port=5  VectorParamsAs1DForOutWhenUnconnected=off
  YAW : Outport  Port=6  VectorParamsAs1DForOutWhenUnconnected=off
  wires:
  x,xdot,xdotdot/1 -> SURGE/1
  y,ydot,ydotdot/1 -> SWAY/1
  z,zdot,zdotdot/1 -> HEAVE/1
  rx,rxdot,rxdotdot/1 -> Radians to Degrees/1
  ry,rydot,rydotdot/1 -> Radians to Degrees1/1
  "rz,rzdot,rzdotdot "/1 -> Radians to Degrees2/1
  6DOF/1 -> rx,rxdot,rxdotdot/1, "rz,rzdot,rzdotdot "/1, ry,rydot,rydotdot/1, y,ydot,ydotdot/1, x,xdot,xdotdot/1, z,zdot,zdotdot/1
  Radians to Degrees/1 -> ROLL/1
  Radians to Degrees1/1 -> PITCH/1
  Radians to Degrees2/1 -> YAW/1

== system SM_Offshore_Windturbine/TOTAL LOADS TO POSITIONS/6 Dof Extractor TO SCOPES  ==
  note: PITCH
  note: HEAVE
  note: SURGE
  6DOF : Inport  PortDimensions=18
  rx,rxdot,rxdotdot : Selector  InputPortWidth=18  IndexOptions=Index vector (dialog)  Indices=[4 10 16]  OutputSizes=1
  ry,rydot,rydotdot : Selector  InputPortWidth=18  IndexOptions=Index vector (dialog)  Indices=[5 11 17]  OutputSizes=1
  "rz,rzdot,rzdotdot " : Selector  InputPortWidth=18  IndexOptions=Index vector (dialog)  Indices=[6 12 18]  OutputSizes=1
  x,xdot,xdotdot : Selector  InputPortWidth=18  IndexOptions=Index vector (dialog)  Indices=[1 7 13]  OutputSizes=1
  y,ydot,ydotdot : Selector  InputPortWidth=18  IndexOptions=Index vector (dialog)  Indices=[2 8 14]  OutputSizes=1
  z,zdot,zdotdot : Selector  InputPortWidth=18  IndexOptions=Index vector (dialog)  Indices=[3 9 15]  OutputSizes=1
  tag scope: HEAVE=global, PITCH=global, ROLL=global, SURGE=global, SWAY=global, YAW=global
  wires:
  x,xdot,xdotdot/1 -> [SURGE]
  y,ydot,ydotdot/1 -> [SWAY]
  z,zdot,zdotdot/1 -> [HEAVE]
  rx,rxdot,rxdotdot/1 -> [ROLL]
  ry,rydot,rydotdot/1 -> [PITCH]
  "rz,rzdot,rzdotdot "/1 -> [YAW]
  6DOF/1 -> rx,rxdot,rxdotdot/1, "rz,rzdot,rzdotdot "/1, ry,rydot,rydotdot/1, y,ydot,ydotdot/1, x,xdot,xdotdot/1, z,zdot,zdotdot/1

== system SM_Offshore_Windturbine/TOTAL LOADS TO POSITIONS/Gravity & Restoring moment ==
  MassMatrix : Inport
  "  " : Selector  NumberOfDimensions=2  InputPortWidth=3  IndexOptions=Index vector (dialog),Index vector (dialog)  Indices=2,6  OutputSizes=1,1
  "     " : Selector  NumberOfDimensions=2  InputPortWidth=3  IndexOptions=Index vector (dialog),Index vector (dialog)  Indices=1,6  OutputSizes=1,1
  Constant : Constant  Value=0
  Constant1 : Constant  Value=[0 0 par.hull.FDA.hydrostatic.Mplat 0 0 0]
  Constant2 : Constant  Value=[0 0 par.hull.FDA.hydrostatic.M 0 0 0]
  Manual Switch : ManualSwitch
  Mux1 : Mux  Inputs=6
  Sum : Sum  Inputs=|+-
  g : Gain  Gain=9.80665
  Gravity & Restoring moment : Outport  VectorParamsAs1DForOutWhenUnconnected=off
  wires:
  Constant2/1 -> Manual Switch/2
  Constant1/1 -> Manual Switch/1
  Manual Switch/1 -> Sum/1
  MassMatrix/1 -> "     "/1, "  "/1
  g/1 -> Gravity & Restoring moment/1
  Sum/1 -> g/1
  Constant/1 -> Mux1/1, Mux1/3, Mux1/6, Mux1/2
  Mux1/1 -> Sum/2
  "     "/1 -> Mux1/4
  "  "/1 -> Mux1/5

== system SM_Offshore_Windturbine/TOTAL LOADS TO POSITIONS/Non linear loads  ==
  MassMatrix : Inport
  hull_speed : Inport  Port=2
  " " : Selector  NumberOfDimensions=2  InputPortWidth=3  IndexOptions=Index vector (dialog),Index vector (dialog)  Indices=3,4  OutputSizes=1,1
  "  " : Selector  NumberOfDimensions=2  InputPortWidth=3  IndexOptions=Index vector (dialog),Index vector (dialog)  Indices=2,6  OutputSizes=1,1
  "   " : Selector  NumberOfDimensions=2  InputPortWidth=3  IndexOptions=Index vector (dialog),Index vector (dialog)  Indices=1,5  OutputSizes=1,1
  "  2" : Selector  NumberOfDimensions=2  InputPortWidth=3  IndexOptions=Index vector (dialog),Index vector (dialog)  Indices=1,1  OutputSizes=1,1
  Cross Product{,1,3..4} (4 alike) : vrlib/Utilities/Cross Product
  Divide : Product  Inputs=/*
  "I extractor " : Selector  NumberOfDimensions=2  InputPortWidth=3  IndexOptions=Index vector (dialog),Index vector (dialog)  Indices=[4 5 6],[4 5 6]  OutputSizes=1,1
  Matrix Multiply1 : Product  Multiplication=Matrix(*)
  Mux : Mux  Inputs=2
  Mux2 : Mux  Inputs=3
  Selector : Selector  InputPortWidth=6  IndexOptions=Index vector (dialog)  Indices=[4 5 6]  OutputSizes=1
  Sum : Sum  Inputs=++|
  Non_linear : Outport  VectorParamsAs1DForOutWhenUnconnected=off
  wires:
  Divide/1 -> Cross Product3/1
  "  2"/1 -> Divide/1  "rcmX"
  Sum/1 -> Mux/2
  Cross Product3/1 -> Sum/1
  Mux/1 -> Non_linear/1
  Mux2/1 -> Cross Product/2, Divide/2
  Cross Product/1 -> Cross Product1/2
  Cross Product1/1 -> Mux/1, Cross Product3/2
  hull_speed/1 -> Selector/1
  " "/1 -> Mux2/2  "rcmY"
  "  "/1 -> Mux2/1  "rcmX"
  "   "/1 -> Mux2/3  "rcmZ"
  MassMatrix/1 -> "I extractor "/1, "   "/1, " "/1, "  "/1, "  2"/1
  "I extractor "/1 -> Matrix Multiply1/1
  Selector/1 -> Cross Product/1, Cross Product4/1, Cross Product1/1, Matrix Multiply1/2  "omega"
  Matrix Multiply1/1 -> Cross Product4/2
  Cross Product4/1 -> Sum/2

== system SM_Offshore_Windturbine/WIND TURBINE/BODIES MOTIONS ==
  Blade Pitch : Inport
  Rotor Torque : Inport  Port=2
  6 DOF : Inport  Port=3
  Control Torque : Inport  Port=4
  1/Idt : Gain  Gain=1/par.WT.prop.Idt
  Integrator : Integrator  InitialCondition=par.IC.wr0*pi/30
  Simscape : Subsystem
  Sum2 : Sum  Inputs=+-|
  Rotor Speed : Outport  VectorParamsAs1DForOutWhenUnconnected=off
  wires:
  Sum2/1 -> 1/Idt/1
  Integrator/1 -> Simscape/1(Omega), Rotor Speed/1
  Rotor Torque/1 -> Sum2/1
  Control Torque/1 -> Sum2/2
  1/Idt/1 -> Integrator/1
  Blade Pitch/1 -> Simscape/2(Blade Pitch)
  6 DOF/1 -> Simscape/3(6 DOF)

== system SM_Offshore_Windturbine/WIND TURBINE/CONTROL SYSTEM ==
  6 DOF : Inport
  Generator speed : Inport  Port=2
  Wind direction : Inport  Port=3
  BLADE PITCH CONTROL : Subsystem
  Low-Pass Filter (Discrete or Continuous) : eeGeneralControl/Low-Pass Filter (Discrete or Continuous)  K=1  T=0.6617  B=inf  A=-inf  init_option=Inherited from block input  x0=0  Ts=-1
  Low-Pass Filter (Discrete or Continuous)1 : eeGeneralControl/Low-Pass Filter (Discrete or Continuous)  K=1  T=10  B=inf  A=-inf  init_option=Inherited from block input  x0=0  Ts=-1
  Manual Switch : ManualSwitch  SampleTime=[0.05, 0]
  Memory : Memory
  TORQUE CONTROL : Subsystem
  YAW CONTROL : ModelReference  ModelNameDialog=YAW_CONTROL.slxp  ModelReferenceVersion=5.20  CopyOfModelProtected=on
  Blade pitch : Outport  VectorParamsAs1DForOutWhenUnconnected=off
  6 DOF nac : Outport  Port=2  VectorParamsAs1DForOutWhenUnconnected=off
  Tg : Outport  Port=3  VectorParamsAs1DForOutWhenUnconnected=off
  tag scope: Speed=global
  wires:
  Generator speed/1 -> [Speed], Low-Pass Filter (Discrete or Continuous)/1
  Low-Pass Filter (Discrete or Continuous)/1 -> BLADE PITCH CONTROL/1(Filtered generator speed), TORQUE CONTROL/1(Filtered generator speed)
  TORQUE CONTROL/1(Generator torque) -> Tg/1
  BLADE PITCH CONTROL/1(Blade pitch) -> TORQUE CONTROL/2(Blade Pitch), Blade pitch/1
  6 DOF/1 -> YAW CONTROL/2, Manual Switch/2
  Manual Switch/1 -> 6 DOF nac/1
  YAW CONTROL/1 -> Manual Switch/1
  Wind direction/1 -> Memory/1
  Memory/1 -> Low-Pass Filter (Discrete or Continuous)1/1
  Low-Pass Filter (Discrete or Continuous)1/1 -> YAW CONTROL/1

== system SM_Offshore_Windturbine/WIND TURBINE/ROTOR LOADS ==
  Blade pitch in : Inport
  Rotor speed : Inport  Port=2
  6 DOF : Inport  Port=3
  Control torque : Inport  Port=4
  Aerodynamic Loads : Subsystem
  Omega to Azimuth : Subsystem
  TowerBaseLoads : Subsystem
  WT Forces : Outport  VectorParamsAs1DForOutWhenUnconnected=off
  RotorTorque : Outport  Port=2  VectorParamsAs1DForOutWhenUnconnected=off
  Wind Direct : Outport  Port=3  VectorParamsAs1DForOutWhenUnconnected=off
  tag scope: ROTTRQ=global, WTFORCES=global
  wires:
  6 DOF/1 -> TowerBaseLoads/1(6 DOF), Aerodynamic Loads/1(6 DOF)
  TowerBaseLoads/1(WTForces) -> [WTFORCES], WT Forces/1
  Aerodynamic Loads/3(AeroLoads) -> TowerBaseLoads/2(AeroLoads)
  Blade pitch in/1 -> Aerodynamic Loads/4(blade pitch)
  Omega to Azimuth/1(Out1) -> Aerodynamic Loads/2(Azimuth)
  Rotor speed/1 -> Aerodynamic Loads/3(Omega), Omega to Azimuth/1(Rotor speed)
  Aerodynamic Loads/2(RotorTorque) -> RotorTorque/1, [ROTTRQ]
  Control torque/1 -> TowerBaseLoads/3(Control torque)
  Aerodynamic Loads/1(Wind Direct) -> Wind Direct/1

== system SM_Offshore_Windturbine/HULL/Viscous loads/Added damping loads ==
  hull_speed : Inport
  " Surge AddDamp" : Gain  Gain=100000
  Constant : Constant  Value=0
  Constant1 : Constant  Value=0
  Heave AddDamp : Gain  Gain=130000
  Mux : Mux  Inputs=6
  Sway AddDamp : Gain  Gain=100000
  Yaw AddDamp : Gain  Gain=13000000
  heave : Selector  InputPortWidth=6  IndexOptions=Index vector (dialog)  Indices=3  OutputSizes=1
  surge : Selector  InputPortWidth=6  IndexOptions=Index vector (dialog)  Indices=1  OutputSizes=1
  sway : Selector  InputPortWidth=6  IndexOptions=Index vector (dialog)  Indices=2  OutputSizes=1
  yaw : Selector  InputPortWidth=6  IndexOptions=Index vector (dialog)  Indices=6  OutputSizes=1
  Added Damping : Outport  VectorParamsAs1DForOutWhenUnconnected=off
  wires:
  Mux/1 -> Added Damping/1
  Heave AddDamp/1 -> Mux/3
  yaw/1 -> Yaw AddDamp/1
  " Surge AddDamp"/1 -> Mux/1
  Sway AddDamp/1 -> Mux/2
  Yaw AddDamp/1 -> Mux/6
  sway/1 -> Sway AddDamp/1
  surge/1 -> " Surge AddDamp"/1
  heave/1 -> Heave AddDamp/1
  hull_speed/1 -> surge/1, sway/1, yaw/1, heave/1
  Constant/1 -> Mux/4
  Constant1/1 -> Mux/5

== system SM_Offshore_Windturbine/HULL/Viscous loads/Subsystem1 ==
  hull_speed : Inport
  hull_position : Inport  Port=2
  " " : Constant  Value=par.wave.velocities.Zrot
  3D rotation matrix : Subsystem
  Clock : Clock
      settings: Decimation=1/par.sym.dt
  Product1 : Product  Multiplication=Matrix(*)
  Subsystem : Subsystem
  Sum1 : Sum  Inputs=-+|
  Sum2 : Sum  Inputs=-+|
  Wave velocities : Subsystem  TreatAsAtomicUnit=on
  rot_speed : Selector  InputPortWidth=6  IndexOptions=Index vector (dialog)  Indices=[4 5 6]  OutputSizes=1
  rx,ry,rz : Selector  InputPortWidth=6  IndexOptions=Index vector (dialog)  Indices=[4 5 6]  OutputSizes=1
  surge : Selector  InputPortWidth=6  IndexOptions=Index vector (dialog)  Indices=1  OutputSizes=1
  sway : Selector  InputPortWidth=6  IndexOptions=Index vector (dialog)  Indices=2  OutputSizes=1
  z : Selector  InputPortWidth=6  IndexOptions=Index vector (dialog)  Indices=3  OutputSizes=1
  Vx : Outport  VectorParamsAs1DForOutWhenUnconnected=off
  Vy : Outport  Port=2  VectorParamsAs1DForOutWhenUnconnected=off
  wires:
  hull_speed/1 -> rot_speed/1, surge/1, sway/1
  rx,ry,rz/1 -> 3D rotation matrix/1(hull_rotation)
  " "/1 -> Product1/2
  3D rotation matrix/1(R(rx,ry,rz)) -> Product1/1
  hull_position/1 -> z/1, rx,ry,rz/1
  Wave velocities/1(Wavex(n)) -> Sum2/2
  surge/1 -> Sum2/1
  Wave velocities/2(Wavey(n)) -> Sum1/2
  Sum1/1 -> Vy/1
  sway/1 -> Sum1/1
  Sum2/1 -> Vx/1
  Product1/1 -> Wave velocities/3(Zrot)
  rot_speed/1 -> Wave velocities/1(hull_rot_speed)
  z/1 -> Wave velocities/2(z_plat)
  Clock/1 -> Subsystem/1(Time)
  Subsystem/1(VxVec) -> Wave velocities/4(VxVec)
  Subsystem/2(VzVec) -> Wave velocities/5(VyVec)
